simulink model "TClabControl_2016a"  (R2016a)
settings: Solver=VariableStepAuto  SolverMode=SingleTasking  StartTime=0.0  StopTime=600  RelTol=1e-3
StartFcn:
  | reset_temp
values from neighbouring files (symbols this model uses):
  P = (K*(1-(s*tau)/2))/((1+(s*tau)/2)*(s+a))    [CA3.m]
  ref = 60 - y_room    (= 37)    [CA3.m]
undefined symbols (not defined in the file or in its folder): yroom
libraries: simulink x2
settings Model: Creator=jamess  LastModifiedBy=jamessaunderson
settings DebuggingCC: SFUnexpectedBacktrackingDiag=error  SFNoUnconditionalDefaultTransitionDiag=error
settings GRTTargetCC: TargetLangStandard=C99 (ISO)
settings ConfigComp: CovMetricSettings=dwe  CovHtmlReporting=off  CovSaveCumulativeToWorkspaceVar=off  CovSaveSingleToWorkspaceVar=off  CovExternalEMLEnable=on

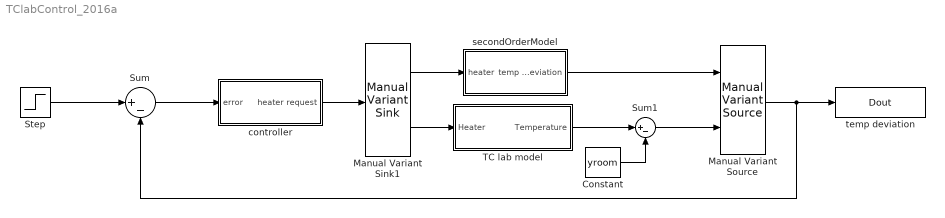
== system TClabControl_2016a ==
  Constant : Constant  Value=yroom
  Manual Variant Sink1 : simulink/Signal Routing/Manual Variant Sink  NumChoices=2  OverrideUsingVariant=V_2
  Manual Variant Source : simulink/Signal Routing/Manual Variant Source  NumChoices=2  OverrideUsingVariant=V_2
  Step : Step  After=ref  SampleTime=0
  Sum : Sum  Inputs=|+-
  Sum1 : Sum  Inputs=|+-
  TC lab model : Subsystem
  controller : Subsystem
  secondOrderModel : Subsystem
  temp deviation : ToWorkspace  VariableName=Dout  SaveFormat=Timeseries  SampleTime=-1
  wires:
  Manual Variant Sink1/2 -> TC lab model/1(Heater)
  secondOrderModel/1(temp deviation) -> Manual Variant Source/1
  Manual Variant Sink1/1 -> secondOrderModel/1(heater)
  controller/1(heater request) -> Manual Variant Sink1/1
  Sum/1 -> controller/1(error)
  Step/1 -> Sum/1
  Manual Variant Source/1 -> temp deviation/1, Sum/2
  TC lab model/1(Temperature) -> Sum1/1
  Sum1/1 -> Manual Variant Source/2
  Constant/1 -> Sum1/2

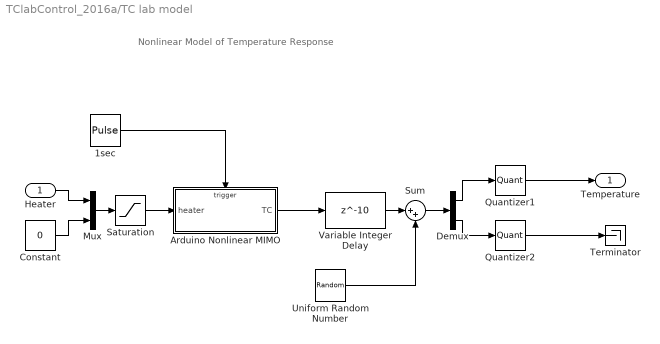
== system TClabControl_2016a/TC lab model ==
  note: Nonlinear Model of Temperature Response
  Heater : Inport
  1sec : DiscretePulseGenerator  PulseType=Time based  Period=1  PulseWidth=50
  Arduino Nonlinear MIMO : Subsystem  TreatAsAtomicUnit=on
  Constant : Constant  Value=0
  Demux : Demux  Outputs=2
  Mux : Mux  Inputs=2
  Quantizer1 : Quantizer
  Quantizer2 : Quantizer
  Saturation : Saturate  UpperLimit=100  LowerLimit=0
  Sum : Sum  Inputs=|++
  Terminator : Terminator
  Uniform Random Number : UniformRandomNumber  Minimum=[-1;-1]  Maximum=[1;1]  SampleTime=1
  Variable Integer Delay : Delay  DelayLength=10  InitialCondition=23  SampleTime=1
  Temperature : Outport
  wires:
  1sec/1 -> Arduino Nonlinear MIMO/Trigger
  Constant/1 -> Mux/2
  Heater/1 -> Mux/1
  Demux/1 -> Quantizer1/1
  Demux/2 -> Quantizer2/1
  Quantizer1/1 -> Temperature/1
  Quantizer2/1 -> Terminator/1
  Arduino Nonlinear MIMO/1(TC) -> Variable Integer Delay/1
  Uniform Random Number/1 -> Sum/2
  Sum/1 -> Demux/1
  Variable Integer Delay/1 -> Sum/1
  Mux/1 -> Saturation/1
  Saturation/1 -> Arduino Nonlinear MIMO/1(heater)

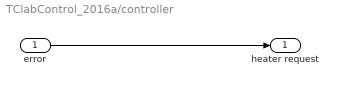
== system TClabControl_2016a/controller ==
  error : Inport
  heater request : Outport
  wires:
  error/1 -> heater request/1

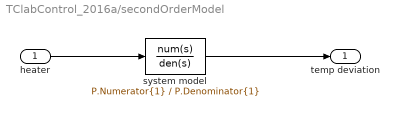
== system TClabControl_2016a/secondOrderModel ==
  heater : Inport
  system model : TransferFcn  Numerator=P.Numerator{1}  Denominator=P.Denominator{1}
  temp deviation : Outport
  wires:
  heater/1 -> system model/1
  system model/1 -> temp deviation/1

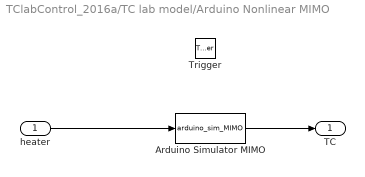
== system TClabControl_2016a/TC lab model/Arduino Nonlinear MIMO ==
  heater : Inport
  Trigger : TriggerPort  VariantControl=Variant
  Arduino Simulator MIMO : MATLABFcn  MATLABFcn=arduino_sim_MIMO
  TC : Outport  InitialOutput=23
  wires:
  Arduino Simulator MIMO/1 -> TC/1
  heater/1 -> Arduino Simulator MIMO/1
